simulink model "uz_drive_model"  (R2021b)
settings: Solver=FixedStepAuto  StartTime=0.0  StopTime=0.6  RelTol=1e-3
PreLoadFcn:
  | uz_pmsm_model_9ph_init_parameter
values from neighbouring files (symbols this model uses):
  c = 2/9*cat(1,tl1,tl2,tl3,tl4,tl5,tl6,tl7,tl8,tl9)    [uz_pmsm_model_9ph_init_parameter.m]
  f_pwm = 50000    [uz_pmsm_model_9ph_init_parameter.m]
  friction_coefficient = 0.001    [uz_pmsm_model_9ph_init_parameter.m]
  inertia = 0.001    [uz_pmsm_model_9ph_init_parameter.m]
  k_i_d = R_1/(2*tau_sum)    (= 78250)    [uz_pmsm_model_9ph_init_parameter.m]
  k_i_q = R_1/(2*tau_sum)    (= 78250)    [uz_pmsm_model_9ph_init_parameter.m]
  k_p_d = L_d/(2*tau_sum)    (= 1250)    [uz_pmsm_model_9ph_init_parameter.m]
  k_p_q = L_q/(2*tau_sum)    (= 1250)    [uz_pmsm_model_9ph_init_parameter.m]
  L_d = 0.5    [uz_pmsm_model_9ph_init_parameter.m]
  L_o1 = Lls    (= 0.08)    [uz_pmsm_model_9ph_init_parameter.m]
  L_o2 = Lls    (= 0.08)    [uz_pmsm_model_9ph_init_parameter.m]
  L_q = 0.5    [uz_pmsm_model_9ph_init_parameter.m]
  L_x1 = Lls    (= 0.08)    [uz_pmsm_model_9ph_init_parameter.m]
  L_x2 = Lls    (= 0.08)    [uz_pmsm_model_9ph_init_parameter.m]
  L_y1 = Lls    (= 0.08)    [uz_pmsm_model_9ph_init_parameter.m]
  L_y2 = Lls    (= 0.08)    [uz_pmsm_model_9ph_init_parameter.m]
  L_zero = Lls    (= 0.08)    [uz_pmsm_model_9ph_init_parameter.m]
  lim_pi = udc/2    (= 280)    [uz_pmsm_model_9ph_init_parameter.m]
  polepair = 2    [uz_pmsm_model_9ph_init_parameter.m]
  psi_pm = 0.6    [uz_pmsm_model_9ph_init_parameter.m]
  R_1 = 31.3    [uz_pmsm_model_9ph_init_parameter.m]
  static_friction_torque = 0.001    [uz_pmsm_model_9ph_init_parameter.m]
  ts = 2/1e6    (= 2e-06)    [uz_pmsm_model_9ph_init_parameter.m]
  udc = 560    [uz_pmsm_model_9ph_init_parameter.m]
undefined symbols (not defined in the file or in its folder): Kpd, Tnd
libraries: nesl_utility x51, fl_lib x43, ee_lib x27, eePwmGeneratorMultilevel x9, simulink x2, slpidlib x2, spsAlphaBetaZerotodq0Lib x1, pid_lib x1, spsdq0toAlphaBetaZeroLib x1
(part 1 of 4)
settings Model: DataTypeOverride=Off  SimulationMode=accelerator  Creator=ts  LastModifiedBy=valen
settings SolverCC: AlgebraicLoopSolver=TrustRegion  AutoInsertRateTranBlk=on
settings DataIOCC: LimitDataPoints=on  SaveOutput=off  SaveTime=off
settings OptimizationCC: BlockReduction=off  ConditionallyExecuteInputs=off  DefaultParameterBehavior=Inlined  LifeSpan=inf
settings DebuggingCC: AlgebraicLoopMsg=error  SingleTaskRateTransMsg=error  AllowSymbolicDim=off  StrictBusMsg=ErrorOnBusTreatedAsVector  SFUnexpectedBacktrackingDiag=warning  SFNoUnconditionalDefaultTransitionDiag=warning  SFExecutionAtInitializationDiag=none  SFMachineParentedDataDiag=warning  ArithmeticOperatorsInVariantConditions=warning
settings HardwareCC: ProdBitPerPointer=32  ProdBitPerSizeT=32  ProdBitPerPtrDiffT=32  ProdLargestAtomicFloat=None  ProdIntDivRoundTo=Undefined  ProdEndianess=Unspecified  ProdWordSize=32  ProdHWDeviceType=ASIC/FPGA->ASIC/FPGA  ProdEqTarget=off
settings SFSimCC: SimUseLocalCustomCode=off  CustomCodeUndefinedFunction=UseInterfaceOnly
settings RTWCC: RTWUseLocalCustomCode=off
settings CodeAppCC: StateflowObjectComments=on
settings GRTTargetCC: TargetLangStandard=C89/C90 (ANSI)
settings ConfigComp: CovScope=ReferencedModels  CovMetricSettings=dw  CovSaveCumulativeToWorkspaceVar=on  CovSaveSingleToWorkspaceVar=on  CovExternalEMLEnable=off  CovSFcnEnable=off

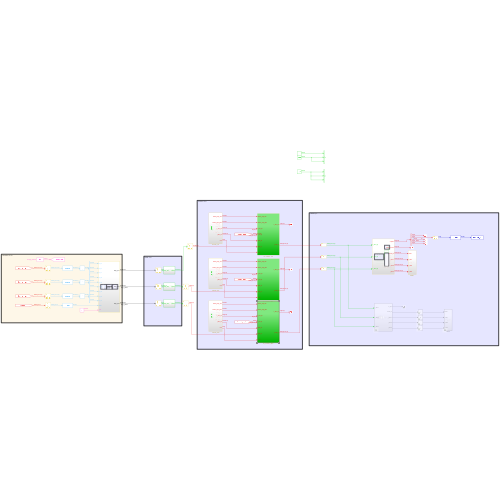
[thumbnail: Simulink's stored preview of the top-level diagram]
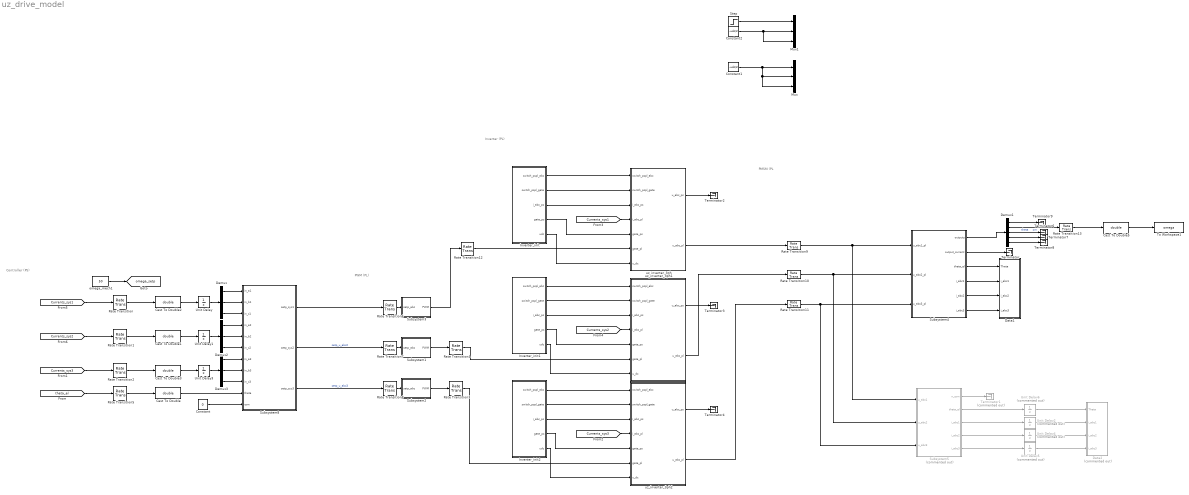
== system uz_drive_model ==
  note: PMSM (PL
  note: Inverter (PL)
  note: PWM (PL)
  note: Controller (PS)
  Cast To Double{,1..3,5} (5 alike) : DataTypeConversion  OutDataTypeStr=double
  Constant : Constant  Value=0
  Constant1 : Constant  Value=-udc/2  SampleTime=ts
  Constant2 : Constant  Value=-udc/2  SampleTime=ts
  Data1 : Subsystem
  Data2 : Subsystem  Commented=on
  Demux : Demux  Outputs=3
  Demux1 : Demux  Outputs=5
  Demux2 : Demux  Outputs=3
  Demux3 : Demux  Outputs=3
  Inverter_init : Subsystem
  Inverter_init1 : Subsystem
  Inverter_init2 : Subsystem
  Mux : Mux  Inputs=3
  Mux1 : Mux  Inputs=3
  Rate Transition{,1..2,5} (4 alike) : RateTransition  OutPortSampleTime=ts_ps
  Rate Transition{6..11} (6 alike) : RateTransition  OutPortSampleTime=ts
  Rate Transition12 : RateTransition  OutPortSampleTime=ts_inv
  Rate Transition13 : RateTransition  OutPortSampleTime=ts_scope
  Rate Transition3 : RateTransition  OutPortSampleTime=ts_inv
  Rate Transition4 : RateTransition  OutPortSampleTime=ts_inv
  Step : Step  Time=0.3  Before=-udc/2  After=udc/2  SampleTime=ts
  Subsystem1 : Subsystem
  Subsystem2 : Subsystem
  Subsystem3 : Subsystem
  Subsystem4 : Subsystem
  Subsystem5 : Subsystem  Commented=on
  Subsystem8 : Subsystem
  Terminator{,2..4,6..9} (8 alike) : Terminator
  Terminator1 : Terminator  Commented=on
  To Workspace1 : ToWorkspace  VariableName=omega  SaveFormat=Timeseries  SampleTime=-1
  Unit Delay : UnitDelay  SampleTime=-1  HasFrameUpgradeWarning=on
  Unit Delay1 : UnitDelay  SampleTime=-1  HasFrameUpgradeWarning=on
  Unit Delay{2,4..6} (4 alike) : UnitDelay  Commented=on  SampleTime=-1  HasFrameUpgradeWarning=on
  Unit Delay3 : UnitDelay  SampleTime=-1  HasFrameUpgradeWarning=on
  omega_mech1 : Constant  Value=50
  uz_inverter_3ph : Subsystem
  uz_inverter_3ph1 : Subsystem
  uz_inverter_3ph2 : Subsystem
  tag scope: omega_setp=global
  wires:
  Unit Delay3/1 -> Demux3/1
  Demux/2 -> Subsystem8/2(in_b1)
  Demux2/1 -> Subsystem8/4(in_a2)
  Demux3/2 -> Subsystem8/8(in_b3)
  Unit Delay1/1 -> Demux2/1
  Demux/3 -> Subsystem8/3(in_c1)
  Demux3/3 -> Subsystem8/9(in_c3)
  Unit Delay/1 -> Demux/1
  Demux3/1 -> Subsystem8/7(in_a3)
  Demux/1 -> Subsystem8/1(in_a1)
  Demux2/2 -> Subsystem8/5(in_b2)
  Demux2/3 -> Subsystem8/6(in_c2)
  Cast To Double/1 -> Subsystem8/10(theta)
  Cast To Double1/1 -> Unit Delay1/1
  Cast To Double2/1 -> Unit Delay/1
  Cast To Double3/1 -> Unit Delay3/1
  Inverter_init/1(switch_pspl_abc) -> uz_inverter_3ph/1(switch_pspl_abc)
  Inverter_init/2(switch_pspl_gate) -> uz_inverter_3ph/2(switch_pspl_gate)
  Inverter_init/3(i_abc_ps) -> uz_inverter_3ph/3(i_abc_ps)
  uz_inverter_3ph/1(u_abc_ps) -> Terminator2/1
  uz_inverter_3ph1/1(u_abc_ps) -> Terminator3/1
  Inverter_init1/4(gate_ps) -> uz_inverter_3ph1/5(gate_ps)
  Inverter_init1/3(i_abc_ps) -> uz_inverter_3ph1/3(i_abc_ps)
  Inverter_init1/2(switch_pspl_gate) -> uz_inverter_3ph1/2(switch_pspl_gate)
  Inverter_init1/1(switch_pspl_abc) -> uz_inverter_3ph1/1(switch_pspl_abc)
  Inverter_init2/1(switch_pspl_abc) -> uz_inverter_3ph2/1(switch_pspl_abc)
  Inverter_init2/2(switch_pspl_gate) -> uz_inverter_3ph2/2(switch_pspl_gate)
  Inverter_init2/3(i_abc_ps) -> uz_inverter_3ph2/3(i_abc_ps)
  Inverter_init2/4(gate_ps) -> uz_inverter_3ph2/5(gate_ps)
  uz_inverter_3ph2/1(u_abc_ps) -> Terminator4/1
  [Currents_sys1] -> uz_inverter_3ph/4(i_abc_pl)
  [Currents_sys2] -> uz_inverter_3ph1/4(i_abc_pl)
  [Currents_sys3] -> uz_inverter_3ph2/4(i_abc_pl)
  Rate Transition/1 -> Cast To Double2/1
  [Currents_sys1] -> Rate Transition/1
  Rate Transition1/1 -> Cast To Double1/1
  [Currents_sys2] -> Rate Transition1/1
  Rate Transition2/1 -> Cast To Double3/1
  [Currents_sys3] -> Rate Transition2/1
  Rate Transition5/1 -> Cast To Double/1
  Constant/1 -> Subsystem8/11(rpm)
  Rate Transition6/1 -> Subsystem3/1(setp_abc)
  Rate Transition7/1 -> Subsystem1/1(setp_abc)
  Rate Transition8/1 -> Subsystem2/1(setp_abc)
  Subsystem4/1(outputs) -> Demux1/1
  Subsystem5/2(theta_el) -> Unit Delay6/1
  Subsystem5/3(i_abc1) -> Unit Delay2/1
  Subsystem5/4(i_abc2) -> Unit Delay4/1
  Subsystem5/5(i_abc3) -> Unit Delay5/1
  Subsystem5/1(n_rpm) -> Terminator1/1
  [theta_el] -> Rate Transition5/1
  Rate Transition9/1 -> Subsystem5/1(u_abc1), Subsystem4/1(u_abc1_pl)
  Rate Transition10/1 -> Subsystem5/2(u_abc2), Subsystem4/2(u_abc2_pl)
  Rate Transition11/1 -> Subsystem5/3(u_abc3), Subsystem4/3(u_abc3_pl)
  Inverter_init/5(udc) -> uz_inverter_3ph/7(u_dc)
  Inverter_init1/5(udc) -> uz_inverter_3ph1/7(u_dc)
  Inverter_init2/5(udc) -> uz_inverter_3ph2/7(u_dc)
  Unit Delay6/1 -> Data2/1(Theta)
  Unit Delay2/1 -> Data2/2(i_abc1)
  Unit Delay4/1 -> Data2/3(i_abc2)
  Unit Delay5/1 -> Data2/4(i_abc3)
  Subsystem4/3(theta_el) -> Data1/1(Theta)
  Subsystem4/4(i_abc1) -> Data1/2(i_abc1)
  Subsystem4/5(i_abc2) -> Data1/3(i_abc2)
  Subsystem4/6(i_abc3) -> Data1/4(i_abc3)
  Rate Transition13/1 -> Cast To Double5/1
  Cast To Double5/1 -> To Workspace1/1
  Demux1/2 -> Rate Transition13/1  "om"
  Demux1/3 -> Terminator6/1  "theta"
  Demux1/4 -> Terminator7/1
  Demux1/5 -> Terminator8/1
  Demux1/1 -> Terminator9/1
  omega_mech1/1 -> [omega_setp]
  Subsystem2/1(PWM) -> Rate Transition3/1
  Subsystem1/1(PWM) -> Rate Transition4/1
  Subsystem3/1(PWM) -> Rate Transition12/1
  Inverter_init/4(gate_ps) -> uz_inverter_3ph/5(gate_ps)
  Subsystem4/2(output_current) -> Terminator/1
  Constant1/1 -> Mux/3, Mux/2, Mux/1
  Constant2/1 -> Mux1/3, Mux1/2
  Step/1 -> Mux1/1
  uz_inverter_3ph/2(u_abc_pl) -> Rate Transition9/1
  uz_inverter_3ph1/2(u_abc_pl) -> Rate Transition10/1
  uz_inverter_3ph2/2(u_abc_pl) -> Rate Transition11/1
  Rate Transition3/1 -> uz_inverter_3ph2/6(gate_pl)
  Rate Transition4/1 -> uz_inverter_3ph1/6(gate_pl)
  Rate Transition12/1 -> uz_inverter_3ph/6(gate_pl)
  Subsystem8/1(setp_sys1) -> Rate Transition6/1
  Subsystem8/2(setp_sys2) -> Rate Transition7/1  "setp_u_abc2"
  Subsystem8/3(setp_sys3) -> Rate Transition8/1  "setp_u_abc3"

== system uz_drive_model/Data1 ==
  Theta : Inport
  i_abc1 : Inport  Port=2
  i_abc2 : Inport  Port=3
  i_abc3 : Inport  Port=4
  Cast To Double4 : DataTypeConversion  OutDataTypeStr=double
  Cast To Double5 : DataTypeConversion  OutDataTypeStr=double
  Cast To Double6 : DataTypeConversion  OutDataTypeStr=double
  Rate Transition12 : RateTransition  OutPortSampleTime=ts_scope
  Rate Transition13 : RateTransition  OutPortSampleTime=ts_scope
  Rate Transition14 : RateTransition  OutPortSampleTime=ts_scope
  Scope : Scope
  To Workspace : ToWorkspace  VariableName=abc1  SaveFormat=Timeseries  SampleTime=-1
  To Workspace1 : ToWorkspace  VariableName=abc2  SaveFormat=Timeseries  SampleTime=-1
  To Workspace2 : ToWorkspace  VariableName=abc3  SaveFormat=Timeseries  SampleTime=-1
  tag scope: Currents_sys1=global, Currents_sys2=global, Currents_sys3=global, theta_el=global
  wires:
  Theta/1 -> [theta_el]
  Cast To Double5/1 -> To Workspace1/1
  i_abc2/1 -> Rate Transition13/1, [Currents_sys2]
  Cast To Double6/1 -> To Workspace2/1
  i_abc3/1 -> Rate Transition14/1, [Currents_sys3]
  Rate Transition14/1 -> Cast To Double6/1
  Rate Transition13/1 -> Cast To Double5/1
  i_abc1/1 -> Rate Transition12/1, [Currents_sys1]
  Cast To Double4/1 -> Scope/1, To Workspace/1
  Rate Transition12/1 -> Cast To Double4/1

== system uz_drive_model/Data2 ==
  Theta : Inport
  i_abc1 : Inport  Port=2
  i_abc2 : Inport  Port=3
  i_abc3 : Inport  Port=4
  Cast To Double4 : DataTypeConversion  OutDataTypeStr=double
  Cast To Double5 : DataTypeConversion  OutDataTypeStr=double
  Cast To Double6 : DataTypeConversion  OutDataTypeStr=double
  Rate Transition12 : RateTransition  OutPortSampleTime=ts_ps
  Rate Transition13 : RateTransition  OutPortSampleTime=ts_ps
  Rate Transition14 : RateTransition  OutPortSampleTime=ts_ps
  Scope : Scope
  To Workspace : ToWorkspace  VariableName=abc1  SaveFormat=Timeseries  SampleTime=-1
  To Workspace1 : ToWorkspace  VariableName=abc2  SaveFormat=Timeseries  SampleTime=-1
  To Workspace2 : ToWorkspace  VariableName=abc3  SaveFormat=Timeseries  SampleTime=-1
  tag scope: Currents_sys1=global, Currents_sys2=global, Currents_sys3=global, theta_el=global
  wires:
  Rate Transition12/1 -> Cast To Double4/1
  Cast To Double4/1 -> To Workspace/1, Scope/1
  i_abc1/1 -> [Currents_sys1], Rate Transition12/1
  Rate Transition13/1 -> Cast To Double5/1
  Rate Transition14/1 -> Cast To Double6/1
  i_abc3/1 -> [Currents_sys3], Rate Transition14/1
  Cast To Double6/1 -> To Workspace2/1
  i_abc2/1 -> [Currents_sys2], Rate Transition13/1
  Cast To Double5/1 -> To Workspace1/1
  Theta/1 -> [theta_el]

== system uz_drive_model/Inverter_init ==
  Constant : Constant  Value=0.0  SampleTime=ts
  Constant1 : Constant  Value=udc
  Constant9 : Constant  Value=false
  Data Type Conversion1 : DataTypeConversion  OutDataTypeStr=boolean  RndMeth=Nearest
  Data Type Conversion2 : DataTypeConversion  OutDataTypeStr=single  RndMeth=Nearest
  Data Type Conversion4 : DataTypeConversion  OutDataTypeStr=boolean
  Data Type Conversion5 : DataTypeConversion  OutDataTypeStr=single  RndMeth=Nearest
  Mux1 : Mux  Inputs=3
  Mux2 : Mux  Inputs=6
  Rate Transition{1..4} (4 alike) : RateTransition  OutPortSampleTime=ts_inv
  switch_pspl_abc : Outport
  switch_pspl_gate : Outport  Port=2
  i_abc_ps : Outport  Port=3
  gate_ps : Outport  Port=4
  udc : Outport  Port=5
  wires:
  Mux2/1 -> Rate Transition3/1
  Data Type Conversion5/1 -> i_abc_ps/1
  Rate Transition1/1 -> Data Type Conversion5/1
  Constant/1 -> Mux2/1, Mux2/3, Mux2/6, Mux2/5, Mux2/4, Mux2/2, Mux1/3, Mux1/2, Mux1/1
  Data Type Conversion1/1 -> gate_ps/1
  Rate Transition4/1 -> switch_pspl_gate/1, switch_pspl_abc/1
  Mux1/1 -> Rate Transition1/1  "Iabc"
  Data Type Conversion4/1 -> Rate Transition4/1
  Constant9/1 -> Data Type Conversion4/1
  Constant1/1 -> Rate Transition2/1
  Rate Transition2/1 -> Data Type Conversion2/1
  Data Type Conversion2/1 -> udc/1
  Rate Transition3/1 -> Data Type Conversion1/1

== system uz_drive_model/Inverter_init1 ==
  Constant : Constant  Value=0.0  SampleTime=ts
  Constant1 : Constant  Value=udc
  Constant9 : Constant  Value=false
  Data Type Conversion1 : DataTypeConversion  OutDataTypeStr=boolean  RndMeth=Nearest
  Data Type Conversion2 : DataTypeConversion  OutDataTypeStr=single  RndMeth=Nearest
  Data Type Conversion4 : DataTypeConversion  OutDataTypeStr=boolean
  Data Type Conversion5 : DataTypeConversion  OutDataTypeStr=single  RndMeth=Nearest
  Mux1 : Mux  Inputs=3
  Mux2 : Mux  Inputs=6
  Rate Transition{1..4} (4 alike) : RateTransition  OutPortSampleTime=ts_inv
  switch_pspl_abc : Outport
  switch_pspl_gate : Outport  Port=2
  i_abc_ps : Outport  Port=3
  gate_ps : Outport  Port=4
  udc : Outport  Port=5
  wires:
  Rate Transition3/1 -> Data Type Conversion1/1
  Data Type Conversion2/1 -> udc/1
  Rate Transition2/1 -> Data Type Conversion2/1
  Constant1/1 -> Rate Transition2/1
  Constant9/1 -> Data Type Conversion4/1
  Data Type Conversion4/1 -> Rate Transition4/1
  Mux1/1 -> Rate Transition1/1  "Iabc"
  Rate Transition4/1 -> switch_pspl_abc/1, switch_pspl_gate/1
  Data Type Conversion1/1 -> gate_ps/1
  Constant/1 -> Mux1/1, Mux1/2, Mux1/3, Mux2/2, Mux2/4, Mux2/5, Mux2/6, Mux2/3, Mux2/1
  Rate Transition1/1 -> Data Type Conversion5/1
  Data Type Conversion5/1 -> i_abc_ps/1
  Mux2/1 -> Rate Transition3/1

== system uz_drive_model/Inverter_init2 ==
  Constant : Constant  Value=0.0  SampleTime=ts
  Constant1 : Constant  Value=udc
  Constant9 : Constant  Value=false
  Data Type Conversion1 : DataTypeConversion  OutDataTypeStr=boolean  RndMeth=Nearest
  Data Type Conversion2 : DataTypeConversion  OutDataTypeStr=single  RndMeth=Nearest
  Data Type Conversion4 : DataTypeConversion  OutDataTypeStr=boolean
  Data Type Conversion5 : DataTypeConversion  OutDataTypeStr=single  RndMeth=Nearest
  Mux1 : Mux  Inputs=3
  Mux2 : Mux  Inputs=6
  Rate Transition{1..4} (4 alike) : RateTransition  OutPortSampleTime=ts_inv
  switch_pspl_abc : Outport
  switch_pspl_gate : Outport  Port=2
  i_abc_ps : Outport  Port=3
  gate_ps : Outport  Port=4
  udc : Outport  Port=5
  wires:
  Mux2/1 -> Rate Transition3/1
  Data Type Conversion5/1 -> i_abc_ps/1
  Rate Transition1/1 -> Data Type Conversion5/1
  Constant/1 -> Mux2/1, Mux2/3, Mux2/6, Mux2/5, Mux2/4, Mux2/2, Mux1/3, Mux1/2, Mux1/1
  Data Type Conversion1/1 -> gate_ps/1
  Rate Transition4/1 -> switch_pspl_gate/1, switch_pspl_abc/1
  Mux1/1 -> Rate Transition1/1  "Iabc"
  Data Type Conversion4/1 -> Rate Transition4/1
  Constant9/1 -> Data Type Conversion4/1
  Constant1/1 -> Rate Transition2/1
  Rate Transition2/1 -> Data Type Conversion2/1
  Data Type Conversion2/1 -> udc/1
  Rate Transition3/1 -> Data Type Conversion1/1

== system uz_drive_model/Subsystem1 ==
  setp_abc : Inport
  Demux : Demux  Outputs=3
  Gain : Gain  Gain=1/(0.5*udc)
  Mux : Mux  Inputs=3
  PWM Generator (Multilevel) : eePwmGeneratorMultilevel/PWM Generator (Multilevel)  topology=Half-bridge  Nsm=1  Tper=1/f_pwm  Ts=ts
      settings: SourceProductBaseCode=PS
  PWM Generator (Multilevel)1 : eePwmGeneratorMultilevel/PWM Generator (Multilevel)  topology=Half-bridge  Nsm=1  Tper=1/f_pwm  Ts=ts
      settings: SourceProductBaseCode=PS
  PWM Generator (Multilevel)2 : eePwmGeneratorMultilevel/PWM Generator (Multilevel)  topology=Half-bridge  Nsm=1  Tper=1/f_pwm  Ts=ts
      settings: SourceProductBaseCode=PS
  PWM : Outport
  wires:
  Gain/1 -> Demux/1
  Mux/1 -> PWM/1
  PWM Generator (Multilevel)2/1 -> Mux/3
  PWM Generator (Multilevel)/1 -> Mux/1
  PWM Generator (Multilevel)1/1 -> Mux/2
  Demux/3 -> PWM Generator (Multilevel)2/1
  Demux/2 -> PWM Generator (Multilevel)1/1
  Demux/1 -> PWM Generator (Multilevel)/1
  setp_abc/1 -> Gain/1

== system uz_drive_model/Subsystem2 ==
  setp_abc : Inport
  Demux : Demux  Outputs=3
  Gain : Gain  Gain=1/(0.5*udc)
  Mux : Mux  Inputs=3
  PWM Generator (Multilevel) : eePwmGeneratorMultilevel/PWM Generator (Multilevel)  topology=Half-bridge  Nsm=1  Tper=1/f_pwm  Ts=ts
      settings: SourceProductBaseCode=PS
  PWM Generator (Multilevel)1 : eePwmGeneratorMultilevel/PWM Generator (Multilevel)  topology=Half-bridge  Nsm=1  Tper=1/f_pwm  Ts=ts
      settings: SourceProductBaseCode=PS
  PWM Generator (Multilevel)2 : eePwmGeneratorMultilevel/PWM Generator (Multilevel)  topology=Half-bridge  Nsm=1  Tper=1/f_pwm  Ts=ts
      settings: SourceProductBaseCode=PS
  PWM : Outport
  wires:
  setp_abc/1 -> Gain/1
  Demux/1 -> PWM Generator (Multilevel)/1
  Demux/2 -> PWM Generator (Multilevel)1/1
  Demux/3 -> PWM Generator (Multilevel)2/1
  PWM Generator (Multilevel)1/1 -> Mux/2
  PWM Generator (Multilevel)/1 -> Mux/1
  PWM Generator (Multilevel)2/1 -> Mux/3
  Mux/1 -> PWM/1
  Gain/1 -> Demux/1

== system uz_drive_model/Subsystem3 ==
  setp_abc : Inport
  Demux : Demux  Outputs=3
  Gain : Gain  Gain=1/(0.5*udc)
  Mux : Mux  Inputs=3
  PWM Generator (Multilevel) : eePwmGeneratorMultilevel/PWM Generator (Multilevel)  topology=Half-bridge  Nsm=1  Tper=1/f_pwm  Ts=ts
      settings: SourceProductBaseCode=PS
  PWM Generator (Multilevel)1 : eePwmGeneratorMultilevel/PWM Generator (Multilevel)  topology=Half-bridge  Nsm=1  Tper=1/f_pwm  Ts=ts
      settings: SourceProductBaseCode=PS
  PWM Generator (Multilevel)2 : eePwmGeneratorMultilevel/PWM Generator (Multilevel)  topology=Half-bridge  Nsm=1  Tper=1/f_pwm  Ts=ts
      settings: SourceProductBaseCode=PS
  PWM : Outport
  wires:
  setp_abc/1 -> Gain/1
  Demux/1 -> PWM Generator (Multilevel)/1
  Demux/2 -> PWM Generator (Multilevel)1/1
  Demux/3 -> PWM Generator (Multilevel)2/1
  PWM Generator (Multilevel)1/1 -> Mux/2
  PWM Generator (Multilevel)/1 -> Mux/1
  PWM Generator (Multilevel)2/1 -> Mux/3
  Mux/1 -> PWM/1
  Gain/1 -> Demux/1

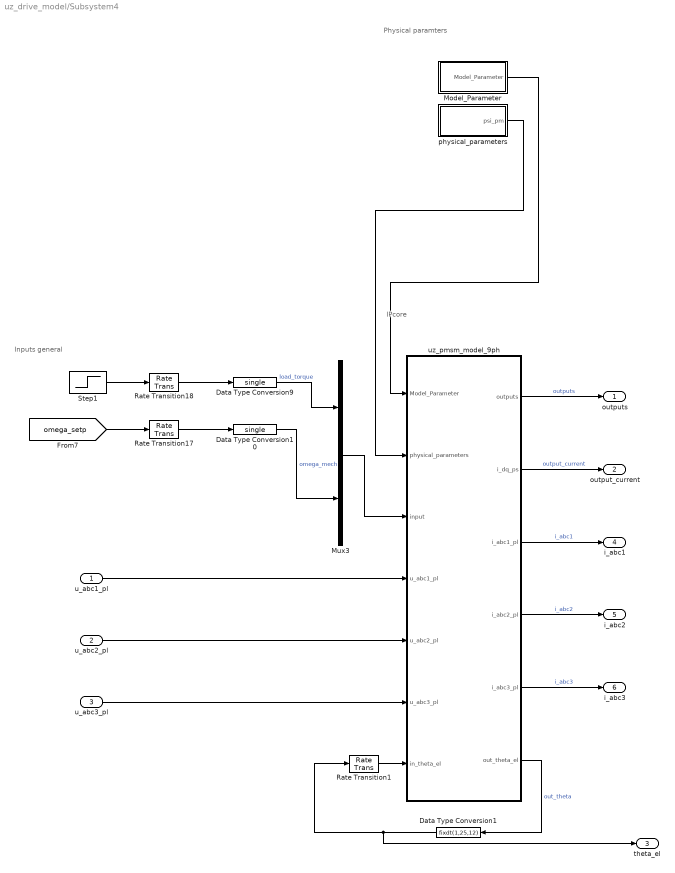
== system uz_drive_model/Subsystem4 ==
  note: IPcore
  note: Physical paramters
  note: Inputs general
  u_abc1_pl : Inport
  u_abc2_pl : Inport  Port=2
  u_abc3_pl : Inport  Port=3
  Data Type Conversion1 : DataTypeConversion  OutDataTypeStr=fixdt(1,25,12)  RndMeth=Nearest
  Data Type Conversion10 : DataTypeConversion  OutDataTypeStr=single  RndMeth=Nearest
  Data Type Conversion9 : DataTypeConversion  OutDataTypeStr=single  RndMeth=Nearest
  Model_Parameter : Subsystem
  Mux3 : Mux  Inputs=2
  Rate Transition1 : RateTransition  OutPortSampleTime=ts
  Rate Transition17 : RateTransition  OutPortSampleTime=ts
  Rate Transition18 : RateTransition  OutPortSampleTime=ts
  Step1 : Step  Time=0.25  After=20  SampleTime=0
  physical_parameters : Subsystem
  uz_pmsm_model_9ph : Subsystem  TreatAsAtomicUnit=on
  outputs : Outport
  output_current : Outport  Port=2
  theta_el : Outport  Port=3
  i_abc1 : Outport  Port=4
  i_abc2 : Outport  Port=5
  i_abc3 : Outport  Port=6
  wires:
  physical_parameters/1(psi_pm) -> uz_pmsm_model_9ph/2(physical_parameters)
  Mux3/1 -> uz_pmsm_model_9ph/3(input)
  u_abc1_pl/1 -> uz_pmsm_model_9ph/4(u_abc1_pl)
  Rate Transition18/1 -> Data Type Conversion9/1
  Data Type Conversion9/1 -> Mux3/1  "load_torque"
  Rate Transition17/1 -> Data Type Conversion10/1
  uz_pmsm_model_9ph/1(outputs) -> outputs/1  "outputs"
  uz_pmsm_model_9ph/6(out_theta_el) -> Data Type Conversion1/1  "out_theta"
  Data Type Conversion10/1 -> Mux3/2  "omega_mech"
  uz_pmsm_model_9ph/5(i_abc3_pl) -> i_abc3/1  "i_abc3"
  Step1/1 -> Rate Transition18/1
  Model_Parameter/1(Model_Parameter) -> uz_pmsm_model_9ph/1(Model_Parameter)
  [omega_setp] -> Rate Transition17/1
  uz_pmsm_model_9ph/3(i_abc1_pl) -> i_abc1/1  "i_abc1"
  uz_pmsm_model_9ph/4(i_abc2_pl) -> i_abc2/1  "i_abc2"
  uz_pmsm_model_9ph/2(i_dq_ps) -> output_current/1  "output_current"
  u_abc3_pl/1 -> uz_pmsm_model_9ph/6(u_abc3_pl)
  u_abc2_pl/1 -> uz_pmsm_model_9ph/5(u_abc2_pl)
  Data Type Conversion1/1 -> Rate Transition1/1, theta_el/1
  Rate Transition1/1 -> uz_pmsm_model_9ph/7(in_theta_el)

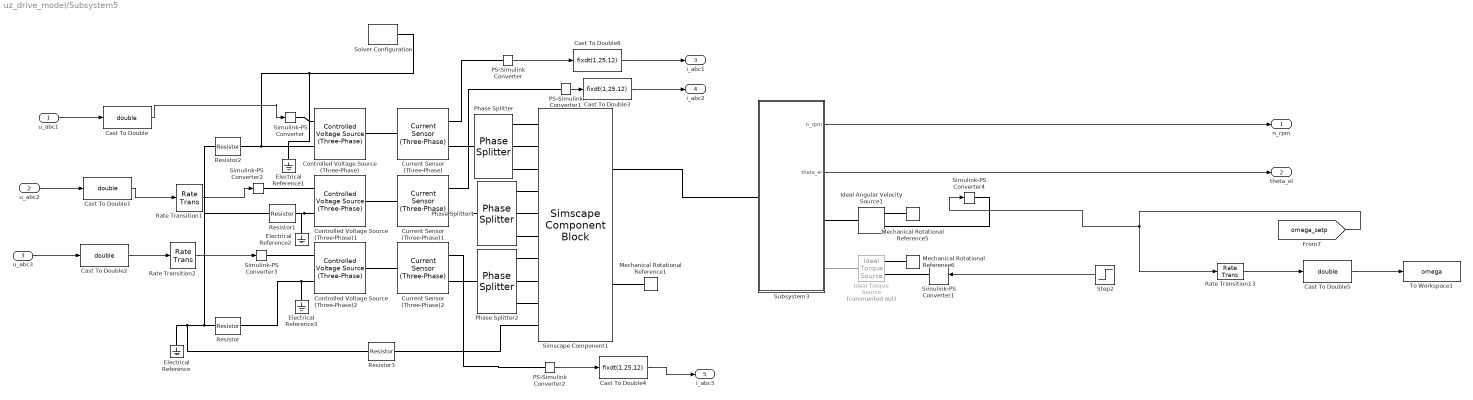
== system uz_drive_model/Subsystem5 ==
  u_abc1 : Inport
  u_abc2 : Inport  Port=2
  u_abc3 : Inport  Port=3
  Cast To Double{,1..2,5} (4 alike) : DataTypeConversion  OutDataTypeStr=double
  Cast To Double3 : DataTypeConversion  OutDataTypeStr=fixdt(1,25,12)
  Cast To Double4 : DataTypeConversion  OutDataTypeStr=fixdt(1,25,12)
  Cast To Double8 : DataTypeConversion  OutDataTypeStr=fixdt(1,25,12)
  Controlled Voltage Source (Three-Phase) : ee_lib/Sources/Controlled Voltage Source (Three-Phase)
      settings: SourceProductBaseCode=PS  InternalSimscapePortConfiguration="{\"Bottom\":[],\"Left\":[{\"id\":\"S\",\"label\":\"S\",\"type\":\"input\"},{\"id\":\"n\",\"label\":\"n\",\"type\":\"foundation.electrical.electrical\"}],\"Right\":[{\"id\":\"N\",\"label\":\"~\",\"type\":\"foundation.electrical.three_phase\"}],\"Top\":[]}"
  Controlled Voltage Source (Three-Phase)1 : ee_lib/Sources/Controlled Voltage Source (Three-Phase)
      settings: SourceProductBaseCode=PS  InternalSimscapePortConfiguration="{\"Bottom\":[],\"Left\":[{\"id\":\"S\",\"label\":\"S\",\"type\":\"input\"},{\"id\":\"n\",\"label\":\"n\",\"type\":\"foundation.electrical.electrical\"}],\"Right\":[{\"id\":\"N\",\"label\":\"~\",\"type\":\"foundation.electrical.three_phase\"}],\"Top\":[]}"
  Controlled Voltage Source (Three-Phase)2 : ee_lib/Sources/Controlled Voltage Source (Three-Phase)
      settings: SourceProductBaseCode=PS  InternalSimscapePortConfiguration="{\"Bottom\":[],\"Left\":[{\"id\":\"S\",\"label\":\"S\",\"type\":\"input\"},{\"id\":\"n\",\"label\":\"n\",\"type\":\"foundation.electrical.electrical\"}],\"Right\":[{\"id\":\"N\",\"label\":\"~\",\"type\":\"foundation.electrical.three_phase\"}],\"Top\":[]}"
  Current Sensor (Three-Phase) : ee_lib/Sensors & Transducers/Current Sensor (Three-Phase)
  Current Sensor (Three-Phase)1 : ee_lib/Sensors & Transducers/Current Sensor (Three-Phase)
  Current Sensor (Three-Phase)2 : ee_lib/Sensors & Transducers/Current Sensor (Three-Phase)
  Electrical Reference{,1..3} (4 alike) : fl_lib/Electrical/Electrical Elements/Electrical Reference
  Ideal Angular Velocity Source1 : fl_lib/Mechanical/Mechanical Sources/Ideal Angular Velocity Source
  Ideal Torque Source : fl_lib/Mechanical/Mechanical Sources/Ideal Torque Source  Commented=on
  Mechanical Rotational Reference1 : fl_lib/Mechanical/Rotational Elements/Mechanical Rotational Reference
  Mechanical Rotational Reference5 : fl_lib/Mechanical/Rotational Elements/Mechanical Rotational Reference
  Mechanical Rotational Reference6 : fl_lib/Mechanical/Rotational Elements/Mechanical Rotational Reference
  PS-Simulink Converter : nesl_utility/PS-Simulink Converter  PhysicalDomain=network_engine_domain  SubClassName=ps_output  LeftPortType=input  RightPortType=output  PseudoPeriodic=off  Frequencies=[]  Unit=inherit  AffineConversion=off
      settings: SourceProductBaseCode=PW,SS
  PS-Simulink Converter1 : nesl_utility/PS-Simulink Converter  PhysicalDomain=network_engine_domain  SubClassName=ps_output  LeftPortType=input  RightPortType=output  PseudoPeriodic=off  Frequencies=[]  Unit=inherit  AffineConversion=off
      settings: SourceProductBaseCode=PW,SS
  PS-Simulink Converter2 : nesl_utility/PS-Simulink Converter  PhysicalDomain=network_engine_domain  SubClassName=ps_output  LeftPortType=input  RightPortType=output  PseudoPeriodic=off  Frequencies=[]  Unit=inherit  AffineConversion=off
      settings: SourceProductBaseCode=PW,SS
  Phase Splitter : ee_lib/Connectors & References/Phase Splitter
      settings: SourceProductBaseCode=PS
  Phase Splitter1 : ee_lib/Connectors & References/Phase Splitter
      settings: SourceProductBaseCode=PS
  Phase Splitter2 : ee_lib/Connectors & References/Phase Splitter
      settings: SourceProductBaseCode=PS
  Rate Transition1 : RateTransition
  Rate Transition13 : RateTransition  OutPortSampleTime=ts_ps
  Rate Transition2 : RateTransition
  Resistor{,1..3} (4 alike) : fl_lib/Electrical/Electrical Elements/Resistor  R=1 MOhm  i_specify=off  i_priority=None  i=0 A  i_nominal_specify=off  i_nominal_unit=A  i_nominal_value=1  v_specify=off  v_priority=None  v=0 V  v_nominal_specify=off  v_nominal_unit=V  v_nominal_value=1
  Simscape Component1 : SimscapeComponentBlock  SourceFile=PMSM_9ph_VSD_Zoric_singleN  ComponentPath=PMSM_9ph_VSD_Zoric_singleN  ComponentVariants="[\"PMSM_9ph_VSD_Zoric_singleN\"]"  ComponentVariantNames="[\"PMSM_9ph_VSD_Zoric_singleN\"]"  ClassName=PMSM_9ph_VSD_Zoric_singleN  SchemaVersion=1  psi_pm=psi_pm Wb  L_d=L_d H  L_q=L_q H  L_0=Lls H  Rs=R_1 Ohm  J=1 kg*m^2  p=polepair  n=9  i_a1_specify=off  i_a1_priority=None  i_a1=0 A  i_a1_nominal_specify=off  i_a1_nominal_unit=A  i_a1_nominal_value=1  i_b1_specify=off  i_b1_priority=None  i_b1=0 A  i_b1_nominal_specify=off  i_b1_nominal_unit=A  i_b1_nominal_value=1  i_c1_specify=off  i_c1_priority=None  i_c1=0 A  i_c1_nominal_specify=off  i_c1_nominal_unit=A  i_c1_nominal_value=1  i_a2_specify=off  i_a2_priority=None  i_a2=0 A  i_a2_nominal_specify=off  i_a2_nominal_unit=A  i_a2_nominal_value=1  i_b2_specify=off  i_b2_priority=None  i_b2=0 A  i_b2_nominal_specify=off  i_b2_nominal_unit=A  i_b2_nominal_value=1  i_c2_specify=off  i_c2_priority=None  i_c2=0 A  i_c2_nominal_specify=off  i_c2_nominal_unit=A  i_c2_nominal_value=1  i_a3_specify=off  i_a3_priority=None  i_a3=0 A  i_a3_nominal_specify=off  i_a3_nominal_unit=A  i_a3_nominal_value=1  i_b3_specify=off  i_b3_priority=None  i_b3=0 A  i_b3_nominal_specify=off  i_b3_nominal_unit=A  i_b3_nominal_value=1  i_c3_specify=off  i_c3_priority=None  i_c3=0 A  i_c3_nominal_specify=off  i_c3_nominal_unit=A  i_c3_nominal_value=1  i_d_specify=off  i_d_priority=None  i_d=0 A  i_d_nominal_specify=off  i_d_nominal_unit=A  i_d_nominal_value=1  i_q_specify=off  i_q_priority=None  i_q=0 A  i_q_nominal_specify=off  i_q_nominal_unit=A  i_q_nominal_value=1  i_a_specify=off  i_a_priority=None  i_a=0 A  i_a_nominal_specify=off  i_a_nominal_unit=A  i_a_nominal_value=1  i_b_specify=off  i_b_priority=None  i_b=0 A  i_b_nominal_specify=off  i_b_nominal_unit=A  i_b_nominal_value=1  i_x1_specify=off  i_x1_priority=None  i_x1=0 A  i_x1_nominal_specify=off  i_x1_nominal_unit=A  i_x1_nominal_value=1  i_y1_specify=off  i_y1_priority=None  i_y1=0 A  i_y1_nominal_specify=off  i_y1_nominal_unit=A  i_y1_nominal_value=1  i_x2_specify=off  i_x2_priority=None  i_x2=0 A  i_x2_nominal_specify=off  i_x2_nominal_unit=A  i_x2_nominal_value=1  i_y2_specify=off  i_y2_priority=None  i_y2=0 A  i_y2_nominal_specify=off  i_y2_nominal_unit=A  i_y2_nominal_value=1  i_x3_specify=off  i_x3_priority=None  i_x3=0 A  i_x3_nominal_specify=off  i_x3_nominal_unit=A  i_x3_nominal_value=1  i_y3_specify=off  i_y3_priority=None  i_y3=0 A  i_y3_nominal_specify=off  i_y3_nominal_unit=A  i_y3_nominal_value=1  i_z_specify=off  i_z_priority=None  i_z=0 A  i_z_nominal_specify=off  i_z_nominal_unit=A  i_z_nominal_value=1  u_d_specify=off  u_d_priority=None  u_d=0 V  u_d_nominal_specify=off  u_d_nominal_unit=V  u_d_nominal_value=1  u_q_specify=off  u_q_priority=None  u_q=0 V  u_q_nominal_specify=off  u_q_nominal_unit=V  u_q_nominal_value=1  u_a_specify=off  u_a_priority=None  u_a=0 V  u_a_nominal_specify=off  u_a_nominal_unit=V  u_a_nominal_value=1  u_b_specify=off  u_b_priority=None  u_b=0 V  u_b_nominal_specify=off  u_b_nominal_unit=V  u_b_nominal_value=1  u_x1_specify=off  u_x1_priority=None  u_x1=0 V  u_x1_nominal_specify=off  u_x1_nominal_unit=V  u_x1_nominal_value=1  u_y1_specify=off  u_y1_priority=None  u_y1=0 V  u_y1_nominal_specify=off  u_y1_nominal_unit=V  u_y1_nominal_value=1  u_x2_specify=off  u_x2_priority=None  u_x2=0 V  u_x2_nominal_specify=off  u_x2_nominal_unit=V  u_x2_nominal_value=1  u_y2_specify=off  u_y2_priority=None  u_y2=0 V  u_y2_nominal_specify=off  u_y2_nominal_unit=V  u_y2_nominal_value=1  u_x3_specify=off  u_x3_priority=None  u_x3=0 V  u_x3_nominal_specify=off  u_x3_nominal_unit=V  u_x3_nominal_value=1  u_y3_specify=off  u_y3_priority=None  u_y3=0 V  u_y3_nominal_specify=off  u_y3_nominal_unit=V  u_y3_nominal_value=1  u_z_specify=off  u_z_priority=None  u_z=0 V  u_z_nominal_specify=off  u_z_nominal_unit=V  u_z_nominal_value=1  m_m_specify=off  m_m_priority=None  m_m=0 N*m  m_m_nominal_specify=off  m_m_nominal_unit=N*m  m_m_nominal_value=1  theta_specify=off  theta_priority=None  theta=0 rad  theta_nominal_specify=off  theta_nominal_unit=rad  theta_nominal_value=1
      settings: CopyFcn=simscape.engine.sli.internal.componentblockcallback(gcbh,'COPY')  PreCopyFcn=simscape.engine.sli.internal.componentblockcallback(gcbh,'PRECOPY')  PreDeleteFcn=simscape.engine.sli.internal.componentblockcallback(gcbh,'PREDELETE')  InternalSimscapePortConfiguration="{\"Bottom\":[],\"Left\":[{\"id\":\"a1\",\"label\":\"a1\",\"type\":\"foundation.electrical.electrical\"},{\"id\":\"b1\",\"label\":\"b1\",\"type\":\"foundation.electrical.electrical\"},{\"id\":\"c1\",\"label\":\"c1\",\"type\":\"foundation.electrical.electrical\"},{\"id\":\"a2\",\"label\":\"a2\",\"type\":\"foundation.electrical.electrical\"},{\"id\":\"b2\",\"label\":\"b2\",\"type\":\"foundation.electrical.electrical\"},{\"id\":\"c2\",\"label\":\"c2\",\"type\":\"foundation.electrical.electrical\"},{\"id\":\"a3\",\"label\":\"a3\",\"type\":\"foundation.electrical.electrical\"},{\"id\":\"b3\",\"label\":\"b3\",\"type\":\"foundation.electrical.electrical\"},{\"id\":\"c3\",\"label\":\"c3\",\"type\":\"foundation.electrical.electrical\"},{\"id\":\"neutral\",\"label\":\"neutral\",\"type\":\"foundation.electrical.electrical\"}],\"Right\":[{\"id\":\"Rot\",\"label\":\"Rot\",\"type\":\"foundation.mechanical.rotational.rotational\"},{\"id\":\"Case\",\"label\":\"Case\",\"type\":\"foundation.mechanical.rotational.rotational\"}],\"Top\":[]}"
      mask Type: Models a 9 phase PMSM with transformation
  Simulink-PS Converter{,2..4} (4 alike) : nesl_utility/Simulink-PS Converter  PhysicalDomain=network_engine_domain  SubClassName=ps_input  LeftPortType=input  RightPortType=output  PseudoPeriodic=off  Frequencies=[]  NoiseDistribution=none  NoiseParameters=[]  Unit=1  AffineConversion=off  FilteringAndDerivatives=provide  SimscapeFilterOrder=1  InputFilterTimeConstant=0.001  UdotUserProvided=0
      settings: SourceProductBaseCode=PW,SS
  Simulink-PS Converter1 : nesl_utility/Simulink-PS Converter  PhysicalDomain=network_engine_domain  SubClassName=ps_input  LeftPortType=input  RightPortType=output  PseudoPeriodic=off  Frequencies=[]  NoiseDistribution=none  NoiseParameters=[]  Unit=1  AffineConversion=off  FilteringAndDerivatives=filter  SimscapeFilterOrder=1  InputFilterTimeConstant=0.001  UdotUserProvided=0
      settings: SourceProductBaseCode=PW,SS
  Solver Configuration : nesl_utility/Solver Configuration  PhysicalDomain=network_engine_domain  SubClassName=solver  LeftPortType=input  RightPortType=generic  Tones=[]  Harmonics=[]  SimulateNoise=off  Profile=off  UseLocalSampling=off  EnableSwitchedLinearOptims=on  FrequencyDomain=off  UseCCode=off  RelTol=0.001  AbsTol=1e-06  MinStep=1e-09  ToWorkspace=off  RevertToSquareIcSolve=off  NumHomotopyIterations=100  PhasorMode=off  PhasorModeNumHarmonics=1  DoDC=off  ResidualTolerance=1e-09  UseLocalSolver=on  LocalSolverChoice=NE_BACKWARD_EULER_ADVANCER  LocalSolverSampleTime=ts  DoFixedCost=on  MaxNonlinIter=3  MaxModeIter=2  ComputeImpulses=off  ImpulseIterations=2  LinearAlgebra=auto  EquationFormulation=NE_TIME_EF  DelaysMemoryBudget=1024  AutomaticFiltering=on  FilteringTimeConstant=0.001  PartitionStorageMethod=AS_NEEDED  PartitionMemoryBudget=1024  PartitionMethod=ROBUST
      settings: SourceProductBaseCode=PW,SS
  Step2 : Step  Time=0.05  After=-1  SampleTime=0
  Subsystem3 : Subsystem
  To Workspace1 : ToWorkspace  VariableName=omega  SaveFormat=Timeseries  SampleTime=-1
  n_rpm : Outport
  theta_el : Outport  Port=2
  i_abc1 : Outport  Port=3
  i_abc2 : Outport  Port=4
  i_abc3 : Outport  Port=5
  wires:
  Step2/1 -> Simulink-PS Converter1/1
  Subsystem3/2(theta_el) -> theta_el/1
  Subsystem3/1(n_rpm) -> n_rpm/1
  u_abc1/1 -> Cast To Double/1
  u_abc2/1 -> Cast To Double1/1
  u_abc3/1 -> Cast To Double2/1
  PS-Simulink Converter/1 -> Cast To Double8/1
  PS-Simulink Converter1/1 -> Cast To Double3/1
  PS-Simulink Converter2/1 -> Cast To Double4/1
  Cast To Double1/1 -> Rate Transition1/1
  Cast To Double8/1 -> i_abc1/1
  Cast To Double3/1 -> i_abc2/1
  Cast To Double4/1 -> i_abc3/1
  Cast To Double/1 -> Simulink-PS Converter/1
  Cast To Double2/1 -> Rate Transition2/1
  Rate Transition2/1 -> Simulink-PS Converter3/1
  Rate Transition1/1 -> Simulink-PS Converter2/1
  [omega_setp] -> Rate Transition13/1, Simulink-PS Converter4/1
  Cast To Double5/1 -> To Workspace1/1
  Rate Transition13/1 -> Cast To Double5/1
  connections:
  Simulink-PS Converter1/RConn1 -- Ideal Torque Source/RConn1
  Subsystem3/RConn1 -- Ideal Angular Velocity Source1/LConn1
  Mechanical Rotational Reference6/LConn1 -- Ideal Torque Source/RConn2
  Mechanical Rotational Reference5/LConn1 -- Ideal Angular Velocity Source1/RConn2
  Ideal Torque Source/LConn1 -- Subsystem3/RConn2
  Simscape Component1/RConn1 -- Subsystem3/LConn1
  Mechanical Rotational Reference1/LConn1 -- Simscape Component1/RConn2
  Phase Splitter/RConn3 -- Simscape Component1/LConn3
  Simscape Component1/LConn2 -- Phase Splitter/RConn2
  Phase Splitter/RConn1 -- Simscape Component1/LConn1
  Simscape Component1/LConn6 -- Phase Splitter1/RConn3
  Simscape Component1/LConn5 -- Phase Splitter1/RConn2
  Simscape Component1/LConn4 -- Phase Splitter1/RConn1
  Simscape Component1/LConn9 -- Phase Splitter2/RConn3
  Simscape Component1/LConn8 -- Phase Splitter2/RConn2
  Simscape Component1/LConn7 -- Phase Splitter2/RConn1
  Current Sensor (Three-Phase)/RConn2 -- Phase Splitter/LConn1
  Controlled Voltage Source (Three-Phase)/RConn1 -- Current Sensor (Three-Phase)/LConn1
  Controlled Voltage Source (Three-Phase)1/RConn1 -- Current Sensor (Three-Phase)1/LConn1
  Current Sensor (Three-Phase)1/RConn2 -- Phase Splitter1/LConn1
  Current Sensor (Three-Phase)2/RConn2 -- Phase Splitter2/LConn1
  Controlled Voltage Source (Three-Phase)2/RConn1 -- Current Sensor (Three-Phase)2/LConn1
  Solver Configuration/RConn1 -- Electrical Reference1/LConn1 -- Resistor2/RConn1 -- Controlled Voltage Source (Three-Phase)/LConn2
  Simulink-PS Converter/RConn1 -- Controlled Voltage Source (Three-Phase)/LConn1
  Simulink-PS Converter2/RConn1 -- Controlled Voltage Source (Three-Phase)1/LConn1
  Controlled Voltage Source (Three-Phase)2/LConn1 -- Simulink-PS Converter3/RConn1
  PS-Simulink Converter/LConn1 -- Current Sensor (Three-Phase)/RConn1
  PS-Simulink Converter1/LConn1 -- Current Sensor (Three-Phase)1/RConn1
  Current Sensor (Three-Phase)2/RConn1 -- PS-Simulink Converter2/LConn1
  Simulink-PS Converter4/RConn1 -- Ideal Angular Velocity Source1/RConn1
  Electrical Reference/LConn1 -- Resistor3/LConn1 -- Resistor2/LConn1 -- Resistor1/LConn1 -- Resistor/LConn1
  Resistor/RConn1 -- Controlled Voltage Source (Three-Phase)2/LConn2 -- Electrical Reference3/LConn1
  Resistor1/RConn1 -- Electrical Reference2/LConn1 -- Controlled Voltage Source (Three-Phase)1/LConn2
  Simscape Component1/LConn10 -- Resistor3/RConn1

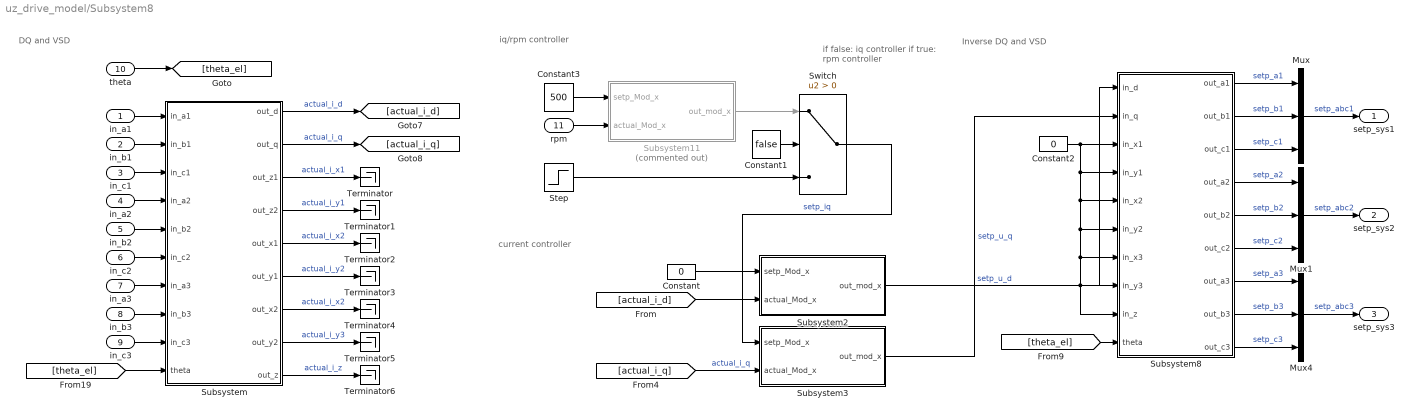
== system uz_drive_model/Subsystem8 ==
  note: DQ and VSD
  note: current controller
  note: iq/rpm controller
  note: if false: iq controller
      | if true: rpm controller
  note: Inverse DQ and VSD
  in_a1 : Inport
  in_b1 : Inport  Port=2
  in_c1 : Inport  Port=3
  in_a2 : Inport  Port=4
  in_b2 : Inport  Port=5
  in_c2 : Inport  Port=6
  in_a3 : Inport  Port=7
  in_b3 : Inport  Port=8
  in_c3 : Inport  Port=9
  theta : Inport  Port=10
  rpm : Inport  Port=11
  Constant : Constant  Value=0
  Constant1 : Constant  Value=false
  Constant2 : Constant  Value=0
  Constant3 : Constant  Value=500
  Mux : Mux  Inputs=3
  Mux1 : Mux  Inputs=3
  Mux4 : Mux  Inputs=3
  Step : Step  Time=0.3  Before=2  After=5  SampleTime=0
  Subsystem : Subsystem
  Subsystem11 : Subsystem  Commented=on
  Subsystem2 : Subsystem
  Subsystem3 : Subsystem
  Subsystem8 : Subsystem
  Switch : Switch  Criteria=u2 > Threshold
  Terminator{,1..6} (7 alike) : Terminator
  setp_sys1 : Outport
  setp_sys2 : Outport  Port=2
  setp_sys3 : Outport  Port=3
  wires:
  Subsystem/4(out_z2) -> Terminator1/1  "actual_i_y1"
  Subsystem8/1(out_a1) -> Mux/1  "setp_a1"
  in_b1/1 -> Subsystem/2(in_b1)
  [theta_el] -> Subsystem8/10(theta)
  Subsystem8/2(out_b1) -> Mux/2  "setp_b1"
  Subsystem8/3(out_c1) -> Mux/3  "setp_c1"
  Subsystem/3(out_z1) -> Terminator/1  "actual_i_x1"
  in_c1/1 -> Subsystem/3(in_c1)
  [actual_i_d] -> Subsystem2/2(actual_Mod_x)
  Constant/1 -> Subsystem2/1(setp_Mod_x)
  Subsystem/6(out_y1) -> Terminator3/1  "actual_i_y2"
  Subsystem/5(out_x1) -> Terminator2/1  "actual_i_x2"
  in_a1/1 -> Subsystem/1(in_a1)
  [actual_i_q] -> Subsystem3/2(actual_Mod_x)  "actual_i_q"
  in_b2/1 -> Subsystem/5(in_b2)
  in_a2/1 -> Subsystem/4(in_a2)
  in_c2/1 -> Subsystem/6(in_c2)
  theta/1 -> [theta_el]
  Mux/1 -> setp_sys1/1  "setp_abc1"
  Subsystem/8(out_y2) -> Terminator5/1  "actual_i_y3"
  Subsystem/7(out_x2) -> Terminator4/1  "actual_i_x2"
  Subsystem/9(out_z) -> Terminator6/1  "actual_i_z"
  in_c3/1 -> Subsystem/9(in_c3)
  in_b3/1 -> Subsystem/8(in_b3)
  in_a3/1 -> Subsystem/7(in_a3)
  Mux1/1 -> setp_sys2/1  "setp_abc2"
  Subsystem8/6(out_c2) -> Mux1/3  "setp_c2"
  Subsystem8/5(out_b2) -> Mux1/2  "setp_b2"
  Subsystem8/4(out_a2) -> Mux1/1  "setp_a2"
  Mux4/1 -> setp_sys3/1  "setp_abc3"
  Subsystem8/7(out_a3) -> Mux4/1  "setp_a3"
  Subsystem8/8(out_b3) -> Mux4/2  "setp_b3"
  Subsystem8/9(out_c3) -> Mux4/3  "setp_c3"
  rpm/1 -> Subsystem11/2(actual_Mod_x)
  Subsystem/1(out_d) -> [actual_i_d]  "actual_i_d"
  Subsystem/2(out_q) -> [actual_i_q]  "actual_i_q"
  [theta_el] -> Subsystem/10(theta)
  Constant2/1 -> Subsystem8/3(in_x1), Subsystem8/8(in_y3), Subsystem8/9(in_z), Subsystem8/7(in_x3), Subsystem8/6(in_y2), Subsystem8/5(in_x2), Subsystem8/4(in_y1)
  Subsystem11/1(out_mod_x) -> Switch/1
  Switch/1 -> Subsystem3/1(setp_Mod_x)  "setp_iq"
  Constant1/1 -> Switch/2
  Step/1 -> Switch/3
  Constant3/1 -> Subsystem11/1(setp_Mod_x)
  Subsystem2/1(out_mod_x) -> Subsystem8/1(in_d)  "setp_u_d"
  Subsystem3/1(out_mod_x) -> Subsystem8/2(in_q)  "setp_u_q"
